simulink model "solar_inverter_2"  (R2023b)
settings: Solver=VariableStepAuto  StartTime=0.0  StopTime=10.0  RelTol=1e-3
libraries: spsMosfetLib x4, spsSeriesRLCBranchLib x1, spsPVArrayLib x1, spspowerguiLib x1, spsVoltageMeasurementLib x1
settings Model: Creator=Vaneebun  LastModifiedBy=visha
settings DebuggingCC: UnconnectedInputMsg=warning  UnconnectedOutputMsg=warning  UnconnectedLineMsg=warning
settings ModelReferenceCC: EnableRefExpFcnMdlSchedulingChecks=on
settings RTWCC: DLArmComputeVersion=19.05

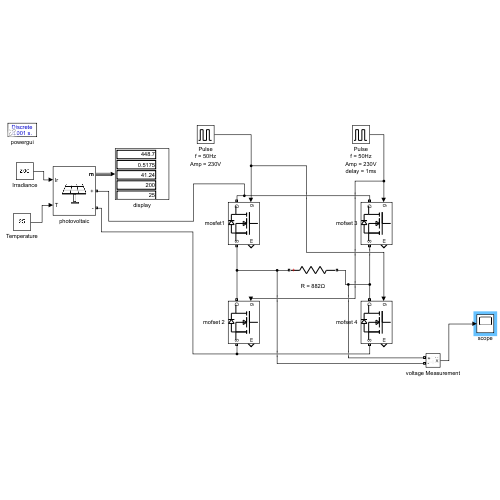
[thumbnail: Simulink's stored preview of the top-level diagram]
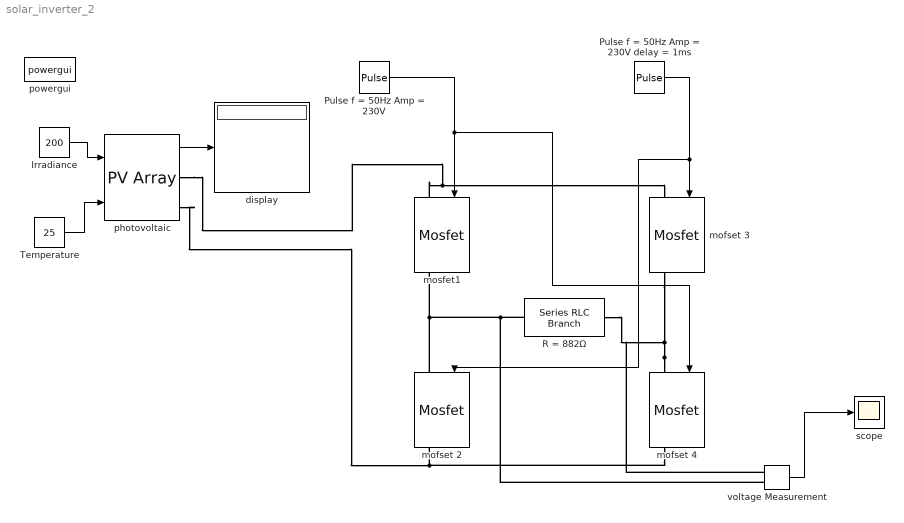
== system solar_inverter_2 ==
  Irradiance : Constant  Value=200
  Pulse f = 50Hz Amp = 230V : DiscretePulseGenerator  PulseType=Time based  Amplitude=230  Period=2e-3  PulseWidth=50
  Pulse f = 50Hz Amp = 230V delay = 1ms : DiscretePulseGenerator  PulseType=Time based  Amplitude=230  Period=2e-3  PulseWidth=50  PhaseDelay=1e-3
  R = 882Ω : spsSeriesRLCBranchLib/Series RLC Branch  LConnTagsString=__new0  RConnTagsString=__new0  BranchType=R  Resistance=882  Inductance=1e-3  SetiL0=off  InitialCurrent=0  Capacitance=1e-6  Setx0=off  InitialVoltage=0  Measurements=Branch voltage and current
  Temperature : Constant  Value=25
  display : Display
  mofset 2 : spsMosfetLib/Mosfet  Ron=0.1  Lon=0  Rd=0.01  Vfd=0  IC=0  Rs=1e5  Cs=inf  Measurements=on
  mofset 3 : spsMosfetLib/Mosfet  Ron=0.1  Lon=0  Rd=0.01  Vfd=0  IC=0  Rs=1e5  Cs=inf  Measurements=on
  mofset 4 : spsMosfetLib/Mosfet  Ron=0.1  Lon=0  Rd=0.01  Vfd=0  IC=0  Rs=1e5  Cs=inf  Measurements=on
  mosfet1 : spsMosfetLib/Mosfet  Ron=0.1  Lon=0  Rd=0.01  Vfd=0  IC=0  Rs=1e5  Cs=inf  Measurements=on
  photovoltaic : spsPVArrayLib/PV Array  Npar=40  Nser=10  PlotType=array @ 1000 W/m2 & specified temperatures  S_vec="[ 1000  500  100 ]"  Temp_C_vec="[ 45 25  ]"  ModuleName=User-defined  PlotWhenSelected=off  Pm=200  Ncell=72  Voc=47.8  Isc=5.4  Vm=40  Im=5  beta_Voc_pc=-0.2984  alpha_Isc_pc=0.046093  beta_Voc=-0.14264  alpha_Isc=0.002489  IL=5.4099  I0=1.6974e-11  nI=0.97696  Rsh=235.9526  Rs=0.43428  RobustModel=off  RobustCellTemperature=313.3991  BAL=off  Tc=1e-6  Tfilter=5e-5
  powergui : spspowerguiLib/powergui  Priority=1  SimulationMode=Discrete  SampleTime=0.001  frequency=60  Iterations=50  frequencyindice=0  Pbase=100e6  ErrMax=1e-4  UnitsV=kV  UnitsW=MW  buscounter=0  FunctionMessages=off  echomessages=off  EnableUseOfTLC=off  CurrentSourceSwitches=off  DisableSnubberDevices=off  DisableRonSwitches=off  DisableVfSwitches=off  DisplayEquations=off  AutomaticDiscreteSolvers=off  SolverType=Tustin/Backward Euler (TBE)  Interpol=off  ExternalGateDelay=off  methode=off  Ts=100  x0status=blocks  SPID=on  SwTol=0  HookPort=off  NonlinearTolerance=1e-4  nMaxIteration=100  ContinueOnMaxIteration=off  RestoreLinks=warning  ResistiveCurrentMeasurement=off  Frange=[0:2:500]  Ylog=off  Xlog=on  ShowGrid=off  save=off  variable=ZData  structure=0  ZoomFFT=off  StartTime=0.0  cycles=1  DisplayStyle=1  fundamental=60  FreqAxis=off  MaxFrequency=1000  frequencyindicesteady=1  RmsSteady=1  display=off
  scope : Scope
  voltage Measurement : spsVoltageMeasurementLib/Voltage Measurement  PhasorSimulation=off  OutputType=Complex  PSBequivalent=0
  wires:
  Irradiance/1 -> photovoltaic/1
  Temperature/1 -> photovoltaic/2
  photovoltaic/1 -> display/1
  voltage Measurement/1 -> scope/1
  Pulse f = 50Hz Amp = 230V/1 -> mosfet1/1, mofset 4/1
  Pulse f = 50Hz Amp = 230V delay = 1ms/1 -> mofset 2/1, mofset 3/1
  connections:
  mosfet1/LConn1 -- mofset 3/LConn1 -- photovoltaic/RConn1
  mofset 4/RConn1 -- photovoltaic/RConn2 -- mofset 2/RConn1
  mofset 4/LConn1 -- mofset 3/RConn1 -- voltage Measurement/LConn1 -- R = 882Ω/RConn1
  R = 882Ω/LConn1 -- voltage Measurement/LConn2 -- mofset 2/LConn1 -- mosfet1/RConn1
